simulink model "HLB_trp"  (R2019b)
settings: Solver=FixedStepDiscrete  StartTime=0.0  StopTime=1000.0  FixedStep=0.01  RelTol=1e-3
InitFcn:
  | %load('20220808.mat')
libraries: driver_model_library x6, simulink x3, CarMaker4SL x1
settings Model: Creator=DOT1BP  LastModifiedBy=DOT1BP
settings ModelReferenceCC: ModelReferenceNumInstancesAllowed=Single

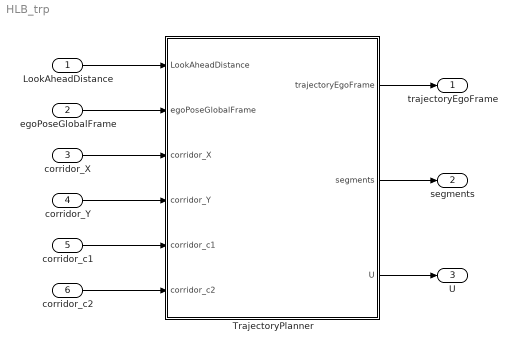
== system HLB_trp ==
  LookAheadDistance : Inport
  egoPoseGlobalFrame : Inport  Port=2  PortDimensions=[3,1]
  corridor_X : Inport  Port=3  PortDimensions=[301,1]
  corridor_Y : Inport  Port=4  PortDimensions=[301,1]
  corridor_c1 : Inport  Port=5  PortDimensions=[301,1]
  corridor_c2 : Inport  Port=6  PortDimensions=[301,1]
  TrajectoryPlanner : Subsystem
  trajectoryEgoFrame : Outport
  segments : Outport  Port=2
  U : Outport  Port=3
  wires:
  TrajectoryPlanner/1(trajectoryEgoFrame) -> trajectoryEgoFrame/1
  TrajectoryPlanner/2(segments) -> segments/1
  TrajectoryPlanner/3(U) -> U/1
  corridor_c2/1 -> TrajectoryPlanner/6(corridor_c2)
  corridor_c1/1 -> TrajectoryPlanner/5(corridor_c1)
  corridor_Y/1 -> TrajectoryPlanner/4(corridor_Y)
  corridor_X/1 -> TrajectoryPlanner/3(corridor_X)
  egoPoseGlobalFrame/1 -> TrajectoryPlanner/2(egoPoseGlobalFrame)
  LookAheadDistance/1 -> TrajectoryPlanner/1("LookAheadDistance ")

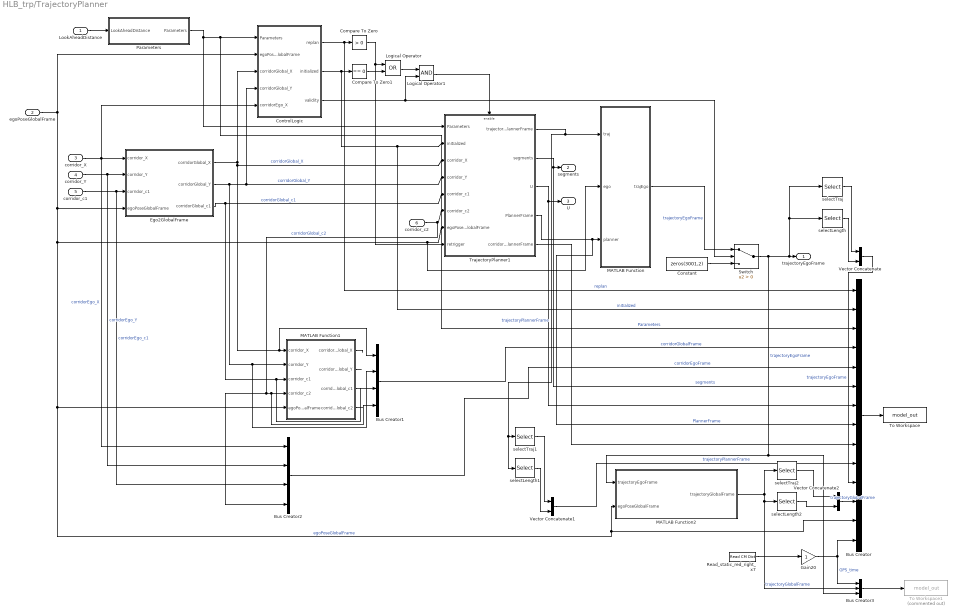
== system HLB_trp/TrajectoryPlanner ==
  "LookAheadDistance " : Inport
  egoPoseGlobalFrame : Inport  Port=2
  corridor_X : Inport  Port=3
  corridor_Y : Inport  Port=4
  corridor_c1 : Inport  Port=5
  corridor_c2 : Inport  Port=6
  Bus Creator : BusCreator  Inputs=14
  Bus Creator1 : BusCreator  Inputs=4
  Bus Creator2 : BusCreator  Inputs=4
  Bus Creator3 : BusCreator  Inputs=3
  Compare To Zero : simulink/Logic and Bit Operations/Compare To Zero  relop=>  OutDataTypeStr=boolean
  Compare To Zero1 : simulink/Logic and Bit Operations/Compare To Zero  relop===  OutDataTypeStr=boolean
  Constant : Constant  Value=zeros(3001,2)
  ControlLogic : Subsystem
  Ego2GlobalFrame : MATLAB Function  TreatAsAtomicUnit=on
  Gain20 : Gain
  Logical Operator : Logic  Operator=OR  AllPortsSameDT=off  OutDataTypeStr=boolean
  Logical Operator1 : Logic  AllPortsSameDT=off  OutDataTypeStr=boolean
  MATLAB Function : MATLAB Function  TreatAsAtomicUnit=on
  MATLAB Function1 : MATLAB Function  TreatAsAtomicUnit=on
  MATLAB Function2 : MATLAB Function  TreatAsAtomicUnit=on
  Parameters : Subsystem
  Read_static_red_right_x7 : CarMaker4SL/Read CM Dict  xname=Time.Global  xsync=off
  Switch : Switch  Criteria=u2 > Threshold
  To Workspace : ToWorkspace  VariableName=model_out  SaveFormat=Timeseries  SampleTime=-1
  To Workspace1 : ToWorkspace  Commented=on  VariableName=model_out  SaveFormat=Timeseries  SampleTime=-1
  TrajectoryPlanner1 : Subsystem
  Vector Concatenate : Concatenate  Mode=Multidimensional array
  Vector Concatenate1 : Concatenate  Mode=Multidimensional array
  Vector Concatenate2 : Concatenate  Mode=Multidimensional array
  selectLength : Selector  NumberOfDimensions=2  InputPortWidth=3  IndexOptions=Index vector (dialog),Index vector (dialog)  Indices=[3001],[1 2]  OutputSizes=1,1
  selectLength1 : Selector  NumberOfDimensions=2  InputPortWidth=3  IndexOptions=Index vector (dialog),Index vector (dialog)  Indices=[3001],[1 2]  OutputSizes=1,1
  selectLength2 : Selector  NumberOfDimensions=2  InputPortWidth=3  IndexOptions=Index vector (dialog),Index vector (dialog)  Indices=[3001],[1 2]  OutputSizes=1,1
  selectTraj : Selector  NumberOfDimensions=2  InputPortWidth=3  IndexOptions=Index vector (dialog),Index vector (dialog)  Indices=linspace(1,300,300),[1 2]  OutputSizes=1,1
  selectTraj1 : Selector  NumberOfDimensions=2  InputPortWidth=3  IndexOptions=Index vector (dialog),Index vector (dialog)  Indices=linspace(1,300,300),[1 2]  OutputSizes=1,1
  selectTraj2 : Selector  NumberOfDimensions=2  InputPortWidth=3  IndexOptions=Index vector (dialog),Index vector (dialog)  Indices=linspace(1,300,300),[1 2]  OutputSizes=1,1
  trajectoryEgoFrame : Outport
  segments : Outport  Port=2
  U : Outport  Port=3
  wires:
  ControlLogic/2(initialized) -> TrajectoryPlanner1/2(initialized), Bus Creator/2, Compare To Zero1/1  "initialized"
  TrajectoryPlanner1/3(U) -> U/1, Bus Creator/7
  Compare To Zero1/1 -> Logical Operator/2
  ControlLogic/1(replan) -> Bus Creator/1, Compare To Zero/1  "replan"
  "LookAheadDistance "/1 -> Parameters/1(LookAheadDistance)
  TrajectoryPlanner1/2(segments) -> Bus Creator/6, segments/1  "segments"
  Compare To Zero/1 -> TrajectoryPlanner1/8(retrigger), Logical Operator/1
  Parameters/1("Parameters ") -> ControlLogic/1(Parameters), Bus Creator/3, TrajectoryPlanner1/1("Parameters ")  "Parameters"
  corridor_c2/1 -> MATLAB Function1/4(corridor_c2), Bus Creator1/4, Bus Creator2/4, TrajectoryPlanner1/6(corridor_c2)  "corridorGlobal_c2"
  MATLAB Function/1(trajEgo) -> Switch/1  "trajectoryEgoFrame"
  TrajectoryPlanner1/1(trajectoryPlannerFrame) -> selectLength1/1, selectTraj1/1, MATLAB Function/1(traj)  "trajectoryPlannerFrame"
  TrajectoryPlanner1/4(PlannerFrame) -> MATLAB Function/3(planner), Bus Creator/8  "PlannerFrame"
  corridor_X/1 -> ControlLogic/5(corridorEgo_X), Ego2GlobalFrame/1(corridor_X), Bus Creator2/1  "corridorEgo_X"
  corridor_Y/1 -> Ego2GlobalFrame/2(corridor_Y), Bus Creator2/2  "corridorEgo_Y"
  corridor_c1/1 -> Bus Creator2/3, Ego2GlobalFrame/3(corridor_c1)  "corridorEgo_c1"
  Ego2GlobalFrame/1(corridorGlobal_X) -> TrajectoryPlanner1/3(corridor_X), Bus Creator1/1, MATLAB Function1/1(corridor_X), ControlLogic/3(corridorGlobal_X)  "corridorGlobal_X"
  Ego2GlobalFrame/2(corridorGlobal_Y) -> MATLAB Function1/2(corridor_Y), Bus Creator1/2, TrajectoryPlanner1/4(corridor_Y), ControlLogic/4(corridorGlobal_Y)  "corridorGlobal_Y"
  Ego2GlobalFrame/3(corridorGlobal_c1) -> MATLAB Function1/3(corridor_c1), Bus Creator1/3, TrajectoryPlanner1/5(corridor_c1)  "corridorGlobal_c1"
  egoPoseGlobalFrame/1 -> ControlLogic/2(egoPoseGlobalFrame), Bus Creator/13, MATLAB Function2/2(egoPoseGlobalFrame), MATLAB Function1/5(egoPoseGlobalFrame), TrajectoryPlanner1/7(egoPoseGlobalFrame), MATLAB Function/2(ego), Ego2GlobalFrame/4(egoPoseGlobalFrame)  "egoPoseGlobalFrame"
  Logical Operator/1 -> Logical Operator1/1
  Logical Operator1/1 -> TrajectoryPlanner1/Enable
  Switch/1 -> selectLength/1, selectTraj/1, trajectoryEgoFrame/1, Bus Creator3/3, MATLAB Function2/1(trajectoryEgoFrame)  "trajectoryEgoFrame"
  Constant/1 -> Switch/3
  Bus Creator/1 -> To Workspace/1
  MATLAB Function1/1(corridorGlobal_X) -> ?
  MATLAB Function1/2(corridorGlobal_Y) -> ?
  MATLAB Function1/3(corridorGlobal_c1) -> ?
  MATLAB Function1/4(corridorGlobal_c2) -> ?
  Bus Creator1/1 -> Bus Creator/4  "corridorGlobalFrame"
  Bus Creator2/1 -> Bus Creator/5  "corridorEgoFrame"
  TrajectoryPlanner1/5(corridorPlannerFrame) -> Bus Creator/9
  MATLAB Function2/1(trajectoryGlobalFrame) -> selectTraj2/1, selectLength2/1, Bus Creator3/2  "trajectoryGlobalFrame"
  Read_static_red_right_x7/1 -> Gain20/1
  Gain20/1 -> Bus Creator/14, Bus Creator3/1  "GPS_time"
  Bus Creator3/1 -> To Workspace1/1
  selectTraj/1 -> Vector Concatenate/1
  selectLength/1 -> Vector Concatenate/2
  ControlLogic/3(validity) -> Logical Operator1/2, Switch/2
  Vector Concatenate/1 -> Bus Creator/11  "trajectoryEgoFrame"
  selectTraj1/1 -> Vector Concatenate1/1
  selectLength1/1 -> Vector Concatenate1/2
  Vector Concatenate1/1 -> Bus Creator/10  "trajectoryPlannerFrame"
  selectTraj2/1 -> Vector Concatenate2/1
  selectLength2/1 -> Vector Concatenate2/2
  Vector Concatenate2/1 -> Bus Creator/12  "trajectoryGlobalFrame"

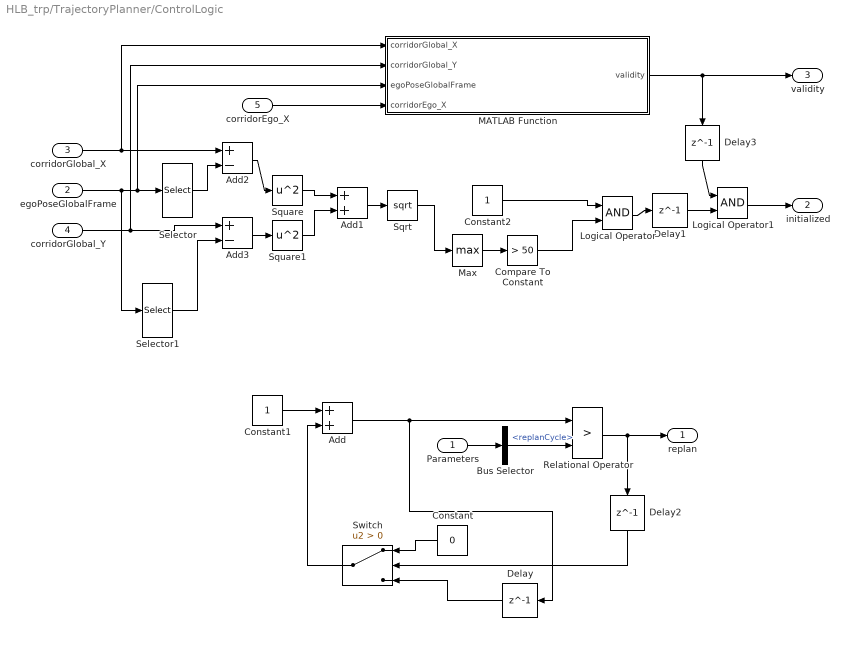
== system HLB_trp/TrajectoryPlanner/ControlLogic ==
  Parameters : Inport
  egoPoseGlobalFrame : Inport  Port=2
  corridorGlobal_X : Inport  Port=3
  corridorGlobal_Y : Inport  Port=4
  corridorEgo_X : Inport  Port=5
  Add : Sum
  Add1 : Sum
  Add2 : Sum  Inputs=+-
  Add3 : Sum  Inputs=+-
  Bus Selector : BusSelector  OutputSignals=replanCycle
  Compare To Constant : simulink/Logic and Bit Operations/Compare To Constant  relop=>  const=50  OutDataTypeStr=boolean
  Constant : Constant  Value=0
  Constant1 : Constant
  Constant2 : Constant
  Delay{,1..3} (4 alike) : Delay  DelayLength=1  InitialCondition=0
  Logical Operator : Logic  AllPortsSameDT=off  OutDataTypeStr=boolean
  Logical Operator1 : Logic  AllPortsSameDT=off  OutDataTypeStr=boolean
  MATLAB Function : MATLAB Function  TreatAsAtomicUnit=on
  Max : MinMax  Function=max
  Relational Operator : RelationalOperator  Operator=>  OutDataTypeStr=boolean  RndMeth=Simplest
  Selector : Selector  InputPortWidth=3  IndexOptions=Index vector (dialog)  Indices=[1]  OutputSizes=1
  Selector1 : Selector  InputPortWidth=3  IndexOptions=Index vector (dialog)  Indices=[2]  OutputSizes=1
  Sqrt : Sqrt  SaturateOnIntegerOverflow=on
  Square : Math  Operator=square  SignedPower=off  SaturateOnIntegerOverflow=on
  Square1 : Math  Operator=square  SignedPower=off  SaturateOnIntegerOverflow=on
  Switch : Switch  Criteria=u2 > Threshold
  replan : Outport
  initialized : Outport  Port=2
  validity : Outport  Port=3
  wires:
  Add/1 -> Relational Operator/1, Delay/1
  Parameters/1 -> Bus Selector/1
  Bus Selector/1 -> Relational Operator/2  "<replanCycle>"
  Relational Operator/1 -> Delay2/1, replan/1
  Constant/1 -> Switch/1
  Delay/1 -> Switch/3
  Switch/1 -> Add/2
  Constant1/1 -> Add/1
  Logical Operator/1 -> Delay1/1
  Constant2/1 -> Logical Operator/1
  Square/1 -> Add1/1
  Square1/1 -> Add1/2
  Add1/1 -> Sqrt/1
  Sqrt/1 -> Max/1
  Compare To Constant/1 -> Logical Operator/2
  Max/1 -> Compare To Constant/1
  Delay2/1 -> Switch/2
  egoPoseGlobalFrame/1 -> Selector/1, MATLAB Function/3(egoPoseGlobalFrame), Selector1/1
  corridorGlobal_X/1 -> Add2/1, MATLAB Function/1(corridorGlobal_X)
  Selector/1 -> Add2/2
  Add2/1 -> Square/1
  Add3/1 -> Square1/1
  corridorGlobal_Y/1 -> Add3/1, MATLAB Function/2(corridorGlobal_Y)
  Selector1/1 -> Add3/2
  MATLAB Function/1(validity) -> Delay3/1, validity/1
  Delay1/1 -> Logical Operator1/2
  Logical Operator1/1 -> initialized/1
  Delay3/1 -> Logical Operator1/1
  corridorEgo_X/1 -> MATLAB Function/4(corridorEgo_X)

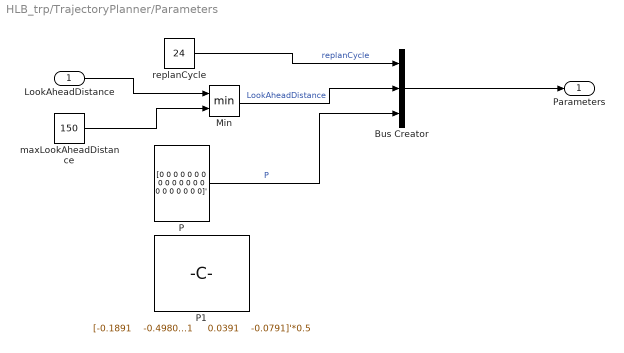
== system HLB_trp/TrajectoryPlanner/Parameters ==
  LookAheadDistance : Inport
  Bus Creator : BusCreator  Inputs=3
  Min : MinMax  Inputs=2
  P : Constant  Value=[0 0 0 0 0 0 0 0 0 0 0 0 0 0 0 0 0 0 0 0 0]'
  P1 : Constant  Value=|
      | [-0.1891
      |    -0.4980
      |     0.6295
      |     0.5723
      |     0.9711
      |    -0.8867
      |    -0.2526
      |    -0.3461
      |     0.3919
      |    -0.0105
      |     0.0010
      |     0.0183
      |     0.0167
      |    -0.0047
      |     0.0494
      |    -0.0250
      |     0.0333
      |    -0.0235
      |     0.0681
      |     0.0391
      |    -0.0791]'*0.5
  maxLookAheadDistance : Constant  Value=150
  replanCycle : Constant  Value=24
  "Parameters " : Outport
  wires:
  Min/1 -> Bus Creator/2  "LookAheadDistance"
  Bus Creator/1 -> "Parameters "/1
  maxLookAheadDistance/1 -> Min/2
  LookAheadDistance/1 -> Min/1
  replanCycle/1 -> Bus Creator/1  "replanCycle"
  P/1 -> Bus Creator/3  "P"

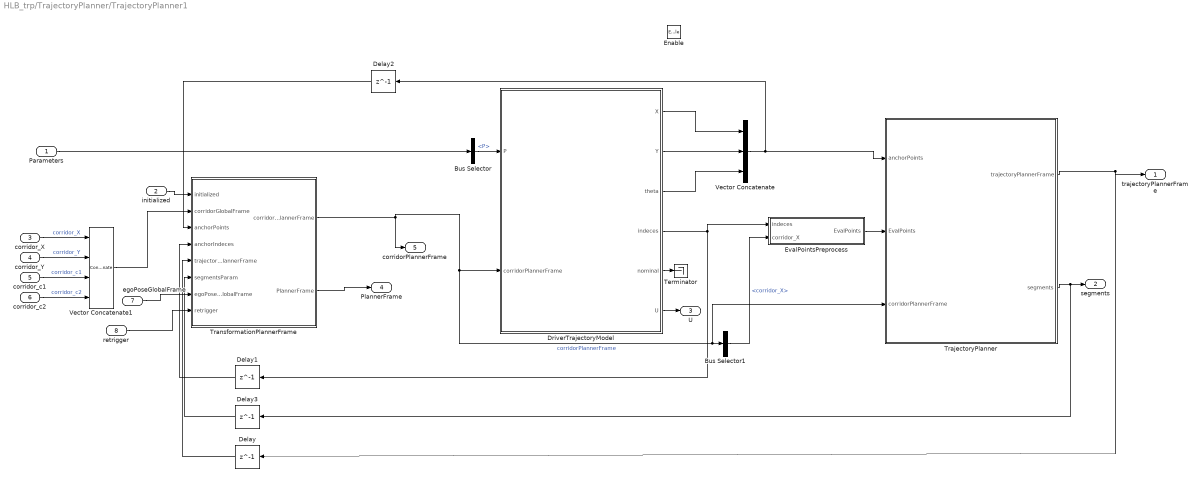
== system HLB_trp/TrajectoryPlanner/TrajectoryPlanner1 ==
  "Parameters " : Inport
  initialized : Inport  Port=2
  corridor_X : Inport  Port=3
  corridor_Y : Inport  Port=4
  corridor_c1 : Inport  Port=5
  corridor_c2 : Inport  Port=6
  egoPoseGlobalFrame : Inport  Port=7
  retrigger : Inport  Port=8
  Enable : EnablePort
  Bus Selector : BusSelector  OutputSignals=P
  Bus Selector1 : BusSelector  OutputSignals=corridor_X
  Delay : Delay  DelayLength=1  InitialCondition=zeros(3001,2)
  Delay1 : Delay  DelayLength=1  InitialCondition=zeros(4,1)
  Delay2 : Delay  DelayLength=1  InitialCondition=zeros(12,1)
  Delay3 : Delay  DelayLength=1  InitialCondition=zeros(3,6)
  DriverTrajectoryModel : Subsystem
  EvalPointsPreprocess : Subsystem
  Terminator : Terminator
  TrajectoryPlanner : Subsystem
  TransformationPlannerFrame : Subsystem
  Vector Concatenate : Concatenate  NumInputs=3
  Vector Concatenate1 : Concatenate  NumInputs=4  Mode=Multidimensional array  ConcatenateDimension=2
  trajectoryPlannerFrame : Outport
  segments : Outport  Port=2
  U : Outport  Port=3
  PlannerFrame : Outport  Port=4
  corridorPlannerFrame : Outport  Port=5
  wires:
  DriverTrajectoryModel/3(theta) -> Vector Concatenate/3
  EvalPointsPreprocess/1(EvalPoints) -> TrajectoryPlanner/2(EvalPoints)
  DriverTrajectoryModel/1(X) -> Vector Concatenate/1
  DriverTrajectoryModel/2(Y) -> Vector Concatenate/2
  DriverTrajectoryModel/5(nominal) -> Terminator/1
  Vector Concatenate/1 -> Delay2/1, TrajectoryPlanner/1(anchorPoints)
  DriverTrajectoryModel/4(indeces) -> Delay1/1, EvalPointsPreprocess/1(indeces)
  TrajectoryPlanner/1(trajectoryPlannerFrame) -> trajectoryPlannerFrame/1, Delay/1
  DriverTrajectoryModel/6(U) -> U/1
  TrajectoryPlanner/2(segments) -> segments/1, Delay3/1
  "Parameters "/1 -> Bus Selector/1
  Bus Selector/1 -> DriverTrajectoryModel/1(P)  "<P>"
  TransformationPlannerFrame/1(corridorPlannerFrame) -> TrajectoryPlanner/3(corridorPlannerFrame), Bus Selector1/1, DriverTrajectoryModel/2(corridorPlannerFrame), corridorPlannerFrame/1  "corridorPlannerFrame"
  initialized/1 -> TransformationPlannerFrame/1(initialized)
  Delay/1 -> TransformationPlannerFrame/5(trajectoryPreviousPlannerFrame)
  corridor_c1/1 -> Vector Concatenate1/3  "corridor_c1"
  corridor_X/1 -> Vector Concatenate1/1  "corridor_X"
  corridor_Y/1 -> Vector Concatenate1/2  "corridor_Y"
  corridor_c2/1 -> Vector Concatenate1/4  "corridor_c2"
  Vector Concatenate1/1 -> TransformationPlannerFrame/2(corridorGlobalFrame)
  Delay1/1 -> TransformationPlannerFrame/4(anchorIndeces)
  Delay2/1 -> TransformationPlannerFrame/3(anchorPoints)
  TransformationPlannerFrame/2(PlannerFrame) -> PlannerFrame/1
  Delay3/1 -> TransformationPlannerFrame/6(segmentsParam)
  egoPoseGlobalFrame/1 -> TransformationPlannerFrame/7(egoPoseGlobalFrame)
  Bus Selector1/1 -> EvalPointsPreprocess/2(corridor_X)  "<corridor_X>"
  retrigger/1 -> TransformationPlannerFrame/8(retrigger)

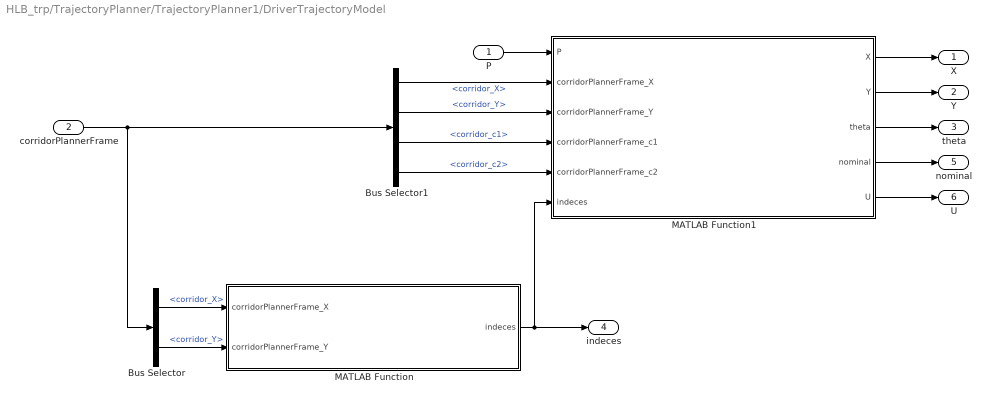
== system HLB_trp/TrajectoryPlanner/TrajectoryPlanner1/DriverTrajectoryModel ==
  P : Inport
  corridorPlannerFrame : Inport  Port=2
  Bus Selector : BusSelector  OutputSignals=corridor_X,corridor_Y
  Bus Selector1 : BusSelector  OutputSignals=corridor_X,corridor_Y,corridor_c1,corridor_c2
  MATLAB Function : MATLAB Function  TreatAsAtomicUnit=on
  MATLAB Function1 : MATLAB Function  TreatAsAtomicUnit=on
  X : Outport
  Y : Outport  Port=2
  theta : Outport  Port=3
  indeces : Outport  Port=4
  nominal : Outport  Port=5
  U : Outport  Port=6
  wires:
  MATLAB Function/1(indeces) -> indeces/1, MATLAB Function1/6(indeces)
  P/1 -> MATLAB Function1/1(P)
  MATLAB Function1/1(X) -> X/1
  MATLAB Function1/2(Y) -> Y/1
  MATLAB Function1/3(theta) -> theta/1
  MATLAB Function1/4(nominal) -> nominal/1
  MATLAB Function1/5(U) -> U/1
  corridorPlannerFrame/1 -> Bus Selector/1, Bus Selector1/1
  Bus Selector/1 -> MATLAB Function/1(corridorPlannerFrame_X)  "<corridor_X>"
  Bus Selector/2 -> MATLAB Function/2(corridorPlannerFrame_Y)  "<corridor_Y>"
  Bus Selector1/1 -> MATLAB Function1/2(corridorPlannerFrame_X)  "<corridor_X>"
  Bus Selector1/2 -> MATLAB Function1/3(corridorPlannerFrame_Y)  "<corridor_Y>"
  Bus Selector1/3 -> MATLAB Function1/4(corridorPlannerFrame_c1)  "<corridor_c1>"
  Bus Selector1/4 -> MATLAB Function1/5(corridorPlannerFrame_c2)  "<corridor_c2>"

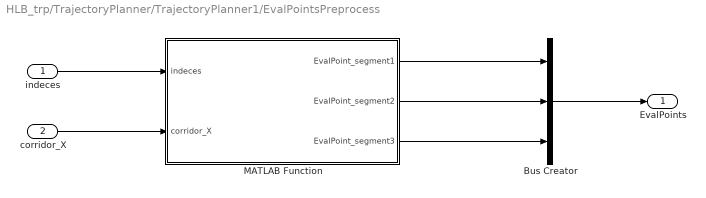
== system HLB_trp/TrajectoryPlanner/TrajectoryPlanner1/EvalPointsPreprocess ==
  indeces : Inport
  corridor_X : Inport  Port=2
  Bus Creator : BusCreator  Inputs=3
  MATLAB Function : MATLAB Function  TreatAsAtomicUnit=on
  EvalPoints : Outport
  wires:
  indeces/1 -> MATLAB Function/1(indeces)
  corridor_X/1 -> MATLAB Function/2(corridor_X)
  MATLAB Function/1(EvalPoint_segment1) -> Bus Creator/1
  MATLAB Function/2(EvalPoint_segment2) -> Bus Creator/2
  MATLAB Function/3(EvalPoint_segment3) -> Bus Creator/3
  Bus Creator/1 -> EvalPoints/1

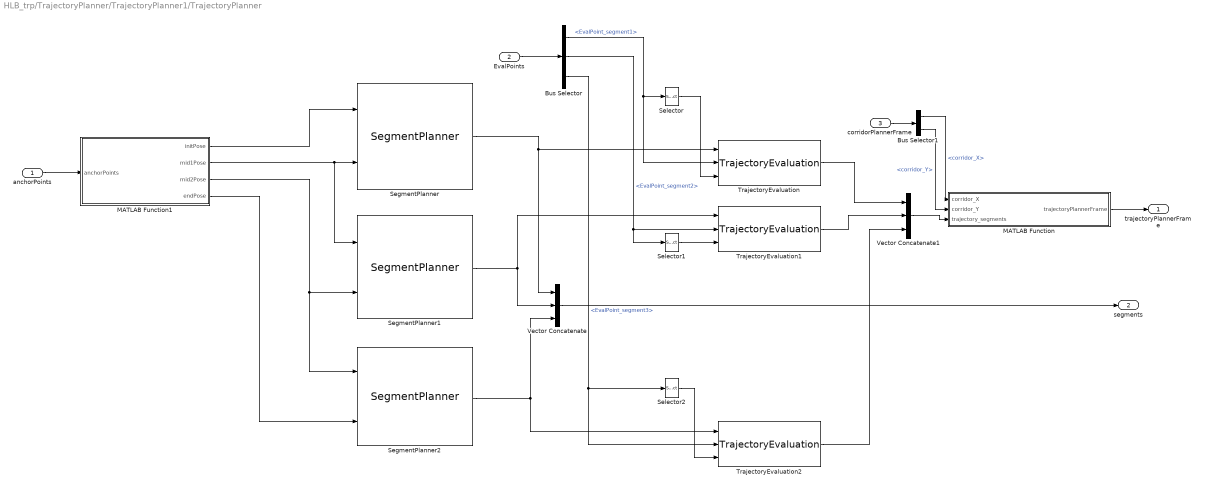
== system HLB_trp/TrajectoryPlanner/TrajectoryPlanner1/TrajectoryPlanner ==
  anchorPoints : Inport
  EvalPoints : Inport  Port=2
  corridorPlannerFrame : Inport  Port=3
  Bus Selector : BusSelector  OutputSignals=EvalPoint_segment1,EvalPoint_segment2,EvalPoint_segment3
  Bus Selector1 : BusSelector  OutputSignals=corridor_X,corridor_Y
  MATLAB Function : MATLAB Function  TreatAsAtomicUnit=on
  MATLAB Function1 : MATLAB Function  TreatAsAtomicUnit=on
  SegmentPlanner : driver_model_library/SegmentPlanner  SystemSampleTime=-1  Latency=0  AutoFrameSizeCalculation=off
  SegmentPlanner1 : driver_model_library/SegmentPlanner  SystemSampleTime=-1  Latency=0  AutoFrameSizeCalculation=off
  SegmentPlanner2 : driver_model_library/SegmentPlanner  SystemSampleTime=-1  Latency=0  AutoFrameSizeCalculation=off
  Selector : Selector  InputPortWidth=1001  IndexOptions=Index vector (dialog)  Indices=1001  OutputSizes=1
  Selector1 : Selector  InputPortWidth=1001  IndexOptions=Index vector (dialog)  Indices=1001  OutputSizes=1
  Selector2 : Selector  InputPortWidth=1001  IndexOptions=Index vector (dialog)  Indices=1001  OutputSizes=1
  TrajectoryEvaluation : driver_model_library/TrajectoryEvaluation  SystemSampleTime=-1  Latency=0  AutoFrameSizeCalculation=off
  TrajectoryEvaluation1 : driver_model_library/TrajectoryEvaluation  SystemSampleTime=-1  Latency=0  AutoFrameSizeCalculation=off
  TrajectoryEvaluation2 : driver_model_library/TrajectoryEvaluation  SystemSampleTime=-1  Latency=0  AutoFrameSizeCalculation=off
  Vector Concatenate : Concatenate  NumInputs=3  Mode=Multidimensional array
  Vector Concatenate1 : Concatenate  NumInputs=3  Mode=Multidimensional array
  trajectoryPlannerFrame : Outport
  segments : Outport  Port=2
  wires:
  anchorPoints/1 -> MATLAB Function1/1(anchorPoints)
  MATLAB Function1/1(initPose) -> SegmentPlanner/1
  MATLAB Function1/2(mid1Pose) -> SegmentPlanner/2, SegmentPlanner1/1
  MATLAB Function1/3(mid2Pose) -> SegmentPlanner1/2, SegmentPlanner2/1
  MATLAB Function1/4(endPose) -> SegmentPlanner2/2
  SegmentPlanner/1 -> TrajectoryEvaluation/1, Vector Concatenate/1
  SegmentPlanner1/1 -> TrajectoryEvaluation1/1, Vector Concatenate/2
  SegmentPlanner2/1 -> Vector Concatenate/3, TrajectoryEvaluation2/1
  Vector Concatenate/1 -> segments/1
  TrajectoryEvaluation/1 -> Vector Concatenate1/1
  TrajectoryEvaluation1/1 -> Vector Concatenate1/2
  TrajectoryEvaluation2/1 -> Vector Concatenate1/3
  EvalPoints/1 -> Bus Selector/1
  Bus Selector/1 -> TrajectoryEvaluation/2, Selector/1  "<EvalPoint_segment1>"
  Bus Selector/2 -> Selector1/1, TrajectoryEvaluation1/2  "<EvalPoint_segment2>"
  Bus Selector/3 -> Selector2/1, TrajectoryEvaluation2/2  "<EvalPoint_segment3>"
  Selector/1 -> TrajectoryEvaluation/3
  Selector1/1 -> TrajectoryEvaluation1/3
  Selector2/1 -> TrajectoryEvaluation2/3
  Vector Concatenate1/1 -> MATLAB Function/3(trajectory_segments)
  MATLAB Function/1(trajectoryPlannerFrame) -> trajectoryPlannerFrame/1
  corridorPlannerFrame/1 -> Bus Selector1/1
  Bus Selector1/2 -> MATLAB Function/2(corridor_Y)  "<corridor_Y>"
  Bus Selector1/1 -> MATLAB Function/1(corridor_X)  "<corridor_X>"

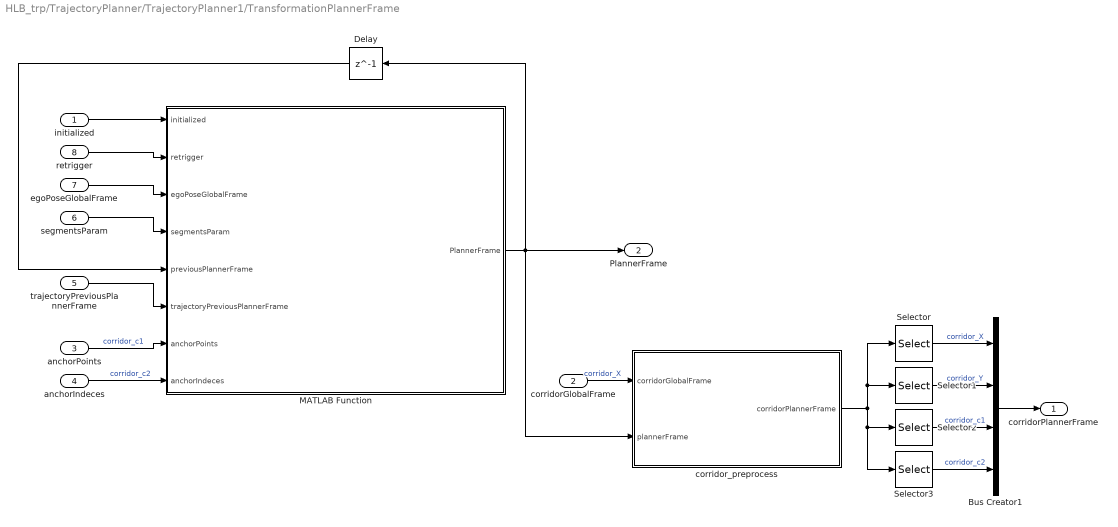
== system HLB_trp/TrajectoryPlanner/TrajectoryPlanner1/TransformationPlannerFrame ==
  initialized : Inport
  corridorGlobalFrame : Inport  Port=2
  anchorPoints : Inport  Port=3
  anchorIndeces : Inport  Port=4
  trajectoryPreviousPlannerFrame : Inport  Port=5
  segmentsParam : Inport  Port=6
  egoPoseGlobalFrame : Inport  Port=7
  retrigger : Inport  Port=8
  Bus Creator1 : BusCreator  Inputs=4
  Delay : Delay  DelayLength=1  InitialCondition=zeros(3,1)
  MATLAB Function : MATLAB Function  TreatAsAtomicUnit=on
  Selector : Selector  NumberOfDimensions=2  InputPortWidth=3  IndexOptions=Select all,Index vector (dialog)  Indices=[1 3],1  OutputSizes=1,1
  Selector1 : Selector  NumberOfDimensions=2  InputPortWidth=3  IndexOptions=Select all,Index vector (dialog)  Indices=[1 3],2  OutputSizes=1,1
  Selector2 : Selector  NumberOfDimensions=2  InputPortWidth=3  IndexOptions=Select all,Index vector (dialog)  Indices=[1 3],3  OutputSizes=1,1
  Selector3 : Selector  NumberOfDimensions=2  InputPortWidth=3  IndexOptions=Select all,Index vector (dialog)  Indices=[1 3],4  OutputSizes=1,1
  corridor_preprocess : MATLAB Function  TreatAsAtomicUnit=on
  corridorPlannerFrame : Outport
  PlannerFrame : Outport  Port=2
  wires:
  Bus Creator1/1 -> corridorPlannerFrame/1
  corridor_preprocess/1(corridorPlannerFrame) -> Selector3/1, Selector2/1, Selector1/1, Selector/1
  Selector/1 -> Bus Creator1/1  "corridor_X"
  Selector1/1 -> Bus Creator1/2  "corridor_Y"
  Selector2/1 -> Bus Creator1/3  "corridor_c1"
  Selector3/1 -> Bus Creator1/4  "corridor_c2"
  trajectoryPreviousPlannerFrame/1 -> MATLAB Function/6(trajectoryPreviousPlannerFrame)
  MATLAB Function/1(PlannerFrame) -> PlannerFrame/1, Delay/1, corridor_preprocess/2(plannerFrame)
  Delay/1 -> MATLAB Function/5(previousPlannerFrame)
  anchorPoints/1 -> MATLAB Function/7(anchorPoints)  "corridor_c1"
  anchorIndeces/1 -> MATLAB Function/8(anchorIndeces)  "corridor_c2"
  corridorGlobalFrame/1 -> corridor_preprocess/1(corridorGlobalFrame)  "corridor_X"
  initialized/1 -> MATLAB Function/1(initialized)
  segmentsParam/1 -> MATLAB Function/4(segmentsParam)
  egoPoseGlobalFrame/1 -> MATLAB Function/3(egoPoseGlobalFrame)
  retrigger/1 -> MATLAB Function/2(retrigger)

== matlab function HLB_trp/TrajectoryPlanner/TrajectoryPlanner1/TrajectoryPlanner/MATLAB Function1 ==
  data: anchorPoints input; initPose output; mid1Pose output; mid2Pose output; endPose output
function [initPose, mid1Pose, mid2Pose, endPose] = preprocess_poses(anchorPoints)

initPose = anchorPoints(1:4:end);
mid1Pose = anchorPoints(2:4:end);
mid2Pose = anchorPoints(3:4:end);
endPose = anchorPoints(4:4:end);

end

== matlab function HLB_trp/TrajectoryPlanner/TrajectoryPlanner1/EvalPointsPreprocess/MATLAB Function ==
  data: indeces input; EvalPoint_segment1 output; corridor_X input; EvalPoint_segment2 output; EvalPoint_segment3 output
function [EvalPoint_segment1, EvalPoint_segment2, EvalPoint_segment3] = selectEvalPoints(indeces, corridor_X)

n_1 = indeces(2) - 1;
n_2 = indeces(3) - indeces(2);
n_3 = indeces(4) - indeces(3) + 1;

EvalPoint_segment1 = zeros(1001,1);
EvalPoint_segment2 = zeros(1001,1);
EvalPoint_segment3 = zeros(1001,1);


EvalPoint_segment1(1:n_1,1) = corridor_X(1:indeces(2)-1,1);
EvalPoint_segment2(1:n_2,1) = corridor_X(indeces(2):indeces(3)-1,1);
EvalPoint_segment3(1:n_3,1) = corridor_X(indeces(3):indeces(4),1);

EvalPoint_segment1(1001,1) = n_1;
EvalPoint_segment2(1001,1) = n_2;
EvalPoint_segment3(1001,1) = n_3;

end

== matlab function HLB_trp/TrajectoryPlanner/TrajectoryPlanner1/DriverTrajectoryModel/MATLAB Function ==
  data: corridorPlannerFrame_X input; indeces output; corridorPlannerFrame_Y input
function indeces  = node_point_model(corridorPlannerFrame_X, corridorPlannerFrame_Y)
% test
n = corridorPlannerFrame_X(301);
corridorPlannerFrame_X = corridorPlannerFrame_X(1:n,1);
corridorPlannerFrame_Y = corridorPlannerFrame_Y(1:n,1);
% delete afterwards
% preprocess bc of test case
non_negative_index = 0;
[non_negative_index] = find(corridorPlannerFrame_X > 0,1);
non_negative_index = non_negative_index(1);
% remove slicing after finished with simulation cases
P = [0; 26.59; 96.91];
n = size(corridorPlannerFrame_X(non_negative_index:end),1);
lengths = zeros(n,1);

lengths(:,1) = (corridorPlannerFrame_X(non_negative_index:end).^2+corridorPlannerFrame_Y(non_negative_index:end).^2).^0.5;

minStepDist = 10; % in meters
indeces = zeros(4,1);
indeces(1) = 1;

L = zeros(1,4);

L(2) = min(lengths(end)-3*minStepDist,max(minStepDist,P(1)));
L(3) = min(lengths(end)-2*minStepDist,max(L(2)+minStepDist,L(2)+P(2)));
L(4) = min(lengths(end)-minStepDist,max(L(3)+minStepDist,L(3)+P(3)));

index_1 = 0;
index_2 = 0;
index_3 = 0;

[index_1] = find(lengths>=L(2),1);
indeces(2) = index_1;
    
[index_2] = find(lengths>=L(3),1);
indeces(3) = index_2;

[index_3] = find(lengths>=L(4),1);
indeces(4) = min(n,index_3);
end

== matlab function HLB_trp/TrajectoryPlanner/TrajectoryPlanner1/DriverTrajectoryModel/MATLAB Function1 ==
  data: P input; X output; corridorPlannerFrame_X input; corridorPlannerFrame_Y input; corridorPlannerFrame_c1 input; corridorPlannerFrame_c2 input; indeces input; Y output; theta output; nominal output; U output
function [X, Y, theta, nominal, U] = driver_model_planner(P, corridorPlannerFrame_X, corridorPlannerFrame_Y, corridorPlannerFrame_c1, corridorPlannerFrame_c2, indeces)
%test
n = corridorPlannerFrame_X(301);
corridorPlannerFrame_X = corridorPlannerFrame_X(1:n,1);
corridorPlannerFrame_Y = corridorPlannerFrame_Y(1:n,1);
corridorPlannerFrame_c1 = corridorPlannerFrame_c1(1:n,1);
corridorPlannerFrame_c2 = corridorPlannerFrame_c2(1:n,1);
%delete afterwards
% preprocess bc of test case
non_negative_index = 0;
[non_negative_index] = find(corridorPlannerFrame_X >= 0,1);
non_negative_index = non_negative_index(1);
corridorPlannerFrame_X = corridorPlannerFrame_X(non_negative_index:end);
corridorPlannerFrame_Y = corridorPlannerFrame_Y(non_negative_index:end);
corridorPlannerFrame_c1 = corridorPlannerFrame_c1(non_negative_index:end);
corridorPlannerFrame_c2 = corridorPlannerFrame_c2(non_negative_index:end);
% remove slicing after finished with simulation cases
P1 = reshape(P(1:21,1),3,7);

X = zeros(4,1);
Y = zeros(4,1);
theta = zeros(4,1);

X_nominal = corridorPlannerFrame_X(indeces);
Y_nominal = corridorPlannerFrame_Y(indeces);
theta_nominal = corridorPlannerFrame_c1(indeces); % orientation in radian
kappa_nominal = zeros(length(indeces)-1, 1);
dkappa_nominal = zeros(length(indeces)-1, 1);

for j=1:length(indeces)-1
    kappa_nominal(j,1) = mean(corridorPlannerFrame_c2(indeces(j):indeces(j+1)));
end

dkappa_vector = zeros(length(corridorPlannerFrame_X),1);
dkappa_vector(2:end) = diff(corridorPlannerFrame_c2)./diff(corridorPlannerFrame_X);
dkappa_vector(1) = diff(corridorPlannerFrame_c2(1:2))/diff(corridorPlannerFrame_X(1:2));
dkappa_vector = movmean(dkappa_vector,50);

% extra corridor information
nominal = [X_nominal; Y_nominal; theta_nominal];

dkappa_nominal = dkappa_vector(indeces);


U = zeros(length(indeces)-1+length(indeces), 1);
U(1:length(indeces)-1,1) = kappa_nominal;
U(length(indeces):end,1) = dkappa_nominal;

% scaling of the predictor variables
kappa_lim = 0.001;
dkappa_lim = 1e-5;
U_lim = [ones(3,1)*kappa_lim; ones(4,1)*dkappa_lim];
U = U./U_lim;

% the ouput of the model is the linear combination of predictor variables
% P parameter matrix is given to the model.
x = P1*U;
x(1:3) = x(1:3);

% the outputs in the local coordinate frame are initialized in [0 0 0],
% therefore their first index is not assigned to anything but kept at zero.
Y(2:4) = Y_nominal(2:4) + x(1:3);
X(2:4) = X_nominal(2:4);
theta(2:4) = atan(tan(theta_nominal(2:4)));

end

== matlab function HLB_trp/TrajectoryPlanner/TrajectoryPlanner1/TrajectoryPlanner/MATLAB Function ==
  data: corridor_X input; corridor_Y input; trajectory_segments input; trajectoryPlannerFrame output
function trajectoryPlannerFrame = trajectoryRearrange(corridor_X, corridor_Y, trajectory_segments)

trajectoryPlannerFrame = zeros(3001,2);

n_1 = trajectory_segments(1001);
n_2 = trajectory_segments(2002);
n_3 = trajectory_segments(3003);

trajectoryPlannerFrame(1:n_1,1) = trajectory_segments(1:n_1,1);
trajectoryPlannerFrame(1:n_1,2) = trajectory_segments(1:n_1,2);
trajectoryPlannerFrame(n_1+1:n_1+n_2,1) = trajectory_segments(1002:1001+n_2,1);
trajectoryPlannerFrame(n_1+1:n_1+n_2,2) = trajectory_segments(1002:1001+n_2,2);
trajectoryPlannerFrame(n_1+n_2+1:n_1+n_2+n_3,1) = trajectory_segments(2003:2002+n_3,1);
trajectoryPlannerFrame(n_1+n_2+1:n_1+n_2+n_3,2) = trajectory_segments(2003:2002+n_3,2);


trajectoryPlannerFrame(3001) = n_1 + n_2 + n_3;

if (any(abs(trajectoryPlannerFrame(1:n_1 + n_2 + n_3,2)-corridor_Y(1:n_1 + n_2 + n_3,1)) > 0.1))
    n_1;
end
end

== matlab function HLB_trp/TrajectoryPlanner/TrajectoryPlanner1/TransformationPlannerFrame/corridor_preprocess ==
  data: corridorGlobalFrame input; corridorPlannerFrame output; plannerFrame input
function corridorPlannerFrame  = corridor_preproc(corridorGlobalFrame, plannerFrame)

% function claculates the corridor coordinates in the current planner coordinate system
% outputs:
%   corridorPlannerFrame
%       corridorPlannerFrameX
%       corridorPlannerFrameY
%       corridorPlannerFrameOrientation
%       corridorPlannerFrameCurvature
% inputs:
%   subsegment - subsegment data (500m segment from the current ego position)
%   deltaPos - X, Y, Theta difference between planner frame and nearest ego
%   point
%
% @copyright (C) 2022 Robert Bosch GmbH.
% The reproduction, distribution and utilization of this file as
% well as the communication of its contents to others without express
% authorization is prohibited. Offenders will be held liable for the
% payment of damages. All rights reserved in the event of the grant
% of a patent, utility model or design.
% @version 0.1
% @date 2022-04-20
corridor = corridorGlobalFrame(:,1:2);
corridorPlannerFrame = zeros(301,4);
n = corridorGlobalFrame(301,1);
corridorPlannerFrame(301,1) = n;

T = [cos(plannerFrame(3)) -sin(plannerFrame(3)); sin(plannerFrame(3)) cos(plannerFrame(3))];
corridorPlannerFrame(1:n,1:2) = ([corridor(1:n,1)-plannerFrame(1) corridor(1:n,2) - plannerFrame(2)])*T;
corridorPlannerFrame(1:n,3) = corridorGlobalFrame(1:n,3) - plannerFrame(3);
corridorPlannerFrame(1:n,4) = corridorGlobalFrame(1:n,4);

end

== matlab function HLB_trp/TrajectoryPlanner/TrajectoryPlanner1/TransformationPlannerFrame/MATLAB Function ==
  data: initialized input; retrigger input; egoPoseGlobalFrame input; segmentsParam input; PlannerFrame output; previousPlannerFrame input; trajectoryPreviousPlannerFrame input; anchorPoints input; anchorIndeces input
function PlannerFrame  = get_planner_frame(initialized, retrigger, egoPoseGlobalFrame, segmentsParam, previousPlannerFrame, trajectoryPreviousPlannerFrame, anchorPoints, anchorIndeces)
% Exceptions: no available points behind the vehicle (at least 2 needed)
% points behind us are way too far from the vehicle
% if delta_x is not monotonously increasing then orientation calc failes
% if delta_x is smaller than 10e-8 consider pi/2 or -pi/2 in case of
% delta_y value


if initialized == 0
    PlannerFrame = egoPoseGlobalFrame;
elseif ~retrigger
    PlannerFrame = previousPlannerFrame;
else
    PlannerFrame = zeros(3,1);
    nbAnchorPoints = floor(size(anchorPoints,1)/3);
    n = trajectoryPreviousPlannerFrame(end,1);
    % finding closest point and getting replanCycle (which point is the new
    % planner frame)
    % transforming trajectory from planner frame to global frame
    T = [cos(previousPlannerFrame(3)) -sin(previousPlannerFrame(3)); sin(previousPlannerFrame(3)) cos(previousPlannerFrame(3))];
    
    trajectoryPreviousGlobalFrame = trajectoryPreviousPlannerFrame(1:end-1,:)*T';
    trajectoryPreviousGlobalFrame(:,1) = trajectoryPreviousGlobalFrame(:,1) + previousPlannerFrame(1);
    trajectoryPreviousGlobalFrame(:,2) = trajectoryPreviousGlobalFrame(:,2) + previousPlannerFrame(2);
    distances = ((trajectoryPreviousGlobalFrame(1:n,1)-egoPoseGlobalFrame(1)).^2 + ...
        (trajectoryPreviousGlobalFrame(1:n,2)-egoPoseGlobalFrame(2)).^2).^0.5;
    replanCycle = find(distances == min(distances),1);
    plannerFrameXInPreviousPlannerFrame = trajectoryPreviousPlannerFrame(replanCycle(1,1), 1);
    plannerFrameYInPreviousPlannerFrame = trajectoryPreviousPlannerFrame(replanCycle(1,1), 2);

    % find the relevant segment
    segment_id = find( anchorPoints > PlannerFrame(1), 1 ) - 1;
    if ((segment_id(1,1)==0) ||(segment_id(1,1) > nbAnchorPoints))
        segment_id = nbAnchorPoints-1;
    end

    % get the parameters of selected segments
    c0_selected = segmentsParam(segment_id(1,1), 4);
    c1_selected = segmentsParam(segment_id(1,1), 5);
    theta_0_selected = anchorPoints(2*nbAnchorPoints + segment_id(1,1));

    % calculate arc length for Theta value of planner point
    s_planner = arc_length(trajectoryPreviousPlannerFrame, anchorIndeces(segment_id(1,1)), replanCycle(1,1));

    % Theta calcuation for planner point
    plannerFrameOrientInPreviousPlannerFrame = theta_0_selected + (c0_selected * s_planner) + ((c1_selected / 2) * s_planner * s_planner);

    T_inv =  [cos(previousPlannerFrame(3)) -sin(previousPlannerFrame(3)); sin(previousPlannerFrame(3)) cos(previousPlannerFrame(3))];

    PlannerFrame(1:2) = (T_inv*[plannerFrameXInPreviousPlannerFrame; plannerFrameYInPreviousPlannerFrame]) + ...
        [previousPlannerFrame(1); previousPlannerFrame(2)];
    PlannerFrame(3) = plannerFrameOrientInPreviousPlannerFrame + previousPlannerFrame(3);

    end

end

function [s] = arc_length(previousTrajectory, startIndex, replanCycle)

dx = diff(previousTrajectory(startIndex:replanCycle,1));
dy = diff(previousTrajectory(startIndex:replanCycle,2));
ds = sqrt(dx.*dx + dy.*dy);
s = sum(ds)*0.7109;

end

== matlab function HLB_trp/TrajectoryPlanner/MATLAB Function ==
  data: traj input; trajEgo output; ego input; planner input
function trajEgo = fcn(traj, ego, planner)
trajEgo = zeros(3001,2);

% trajPlanner to trajGlobal
n = traj(3001,1);
trajGlobal = zeros(n,2);
T = [cos(planner(3)) -sin(planner(3)); sin(planner(3)) cos(planner(3))];
trajGlobal(:,:) = [traj(1:n,:)*T'] + [ones(n,1)*planner(1) ones(n,1)*planner(2)];

% trajGlobal to trajEgo
T = [cos(ego(3)) sin(ego(3)); -sin(ego(3)) cos(ego(3))];
trajEgo(1:n,:) = (trajGlobal - [ones(n,1)*ego(1) ones(n,1)*ego(2)])*T';
trajEgo(3001,1) = n;

== matlab function HLB_trp/TrajectoryPlanner/Ego2GlobalFrame ==
  data: corridor_X input; corridorGlobal_X output; corridor_Y input; corridor_c1 input; egoPoseGlobalFrame input; corridorGlobal_Y output; corridorGlobal_c1 output
function [corridorGlobal_X, corridorGlobal_Y, corridorGlobal_c1] = fcn(corridor_X, corridor_Y, corridor_c1, egoPoseGlobalFrame)

    n=corridor_X(301,1);
    corridorGlobal_X = zeros(301,1);
    corridorGlobal_Y = zeros(301,1);
    corridorGlobal_c1 = zeros(301,1);
    corridorGlobal = zeros(301,2);

    T = [cos(egoPoseGlobalFrame(3)) -sin(egoPoseGlobalFrame(3)); sin(egoPoseGlobalFrame(3)) cos(egoPoseGlobalFrame(3))];
    corridorGlobal(1:n,:) = [corridor_X(1:n,1) corridor_Y(1:n,1)]*T' + [ones(n,1)*egoPoseGlobalFrame(1) ones(n,1)*egoPoseGlobalFrame(2)];

    corridorGlobal_X(1:n,1) = corridorGlobal(1:n,1);
    corridorGlobal_Y(1:n,1) = corridorGlobal(1:n,2);
    corridorGlobal_c1(1:n,1) = corridor_c1(1:n,1) + egoPoseGlobalFrame(3);
    
    corridorGlobal_X(301,1) = n;
    corridorGlobal_Y(301,1) = n;
    corridorGlobal_c1(301,1) = n;

end

== matlab function HLB_trp/TrajectoryPlanner/ControlLogic/MATLAB Function ==
  data: corridorGlobal_X input; corridorGlobal_Y input; validity output; egoPoseGlobalFrame input; corridorEgo_X input
function validity = corridorValidity(corridorGlobal_X, corridorGlobal_Y, egoPoseGlobalFrame, corridorEgo_X)

n = corridorGlobal_X(301);
distances = ((corridorGlobal_X(1:n) - egoPoseGlobalFrame(1)).^2 + (corridorGlobal_Y(1:n) - egoPoseGlobalFrame(2)).^2).^0.5;
[invalid_idx] = find(abs(diff(distances)) > 6, 1);

distance_first_point = ((corridorGlobal_X(1) - egoPoseGlobalFrame(1))^2 + (corridorGlobal_Y(1) - egoPoseGlobalFrame(2))^2)^0.5;

% checking monotonity, number of corridor points, distance of first point,
% distance between adjacent points
if ~isempty(invalid_idx) ||  distance_first_point > 5 || ~all(diff(corridorEgo_X(1:n))>0) || n < 2
    validity = false;
else
    validity = true;
end

end

== matlab function HLB_trp/TrajectoryPlanner/MATLAB Function1 ==
  data: corridor_X input; corridorGlobal_X output; corridor_Y input; corridor_c1 input; corridor_c2 input; egoPoseGlobalFrame input; corridorGlobal_Y output; corridorGlobal_c1 output; corridorGlobal_c2 output
function [corridorGlobal_X, corridorGlobal_Y, corridorGlobal_c1, corridorGlobal_c2] = fcn(corridor_X, corridor_Y, corridor_c1, corridor_c2, egoPoseGlobalFrame)

n = corridor_X(301);

if (n >= 2)
    distances_vec = ((corridor_X(1:n) - egoPoseGlobalFrame(1)).^2 + (corridor_Y(1:n) - egoPoseGlobalFrame(2)).^2).^0.5;
    [closest_point_index] = find(distances_vec == min(distances_vec),1);
    closest_point_index = closest_point_index(1);

    corridorGlobal_X = corridor_X(closest_point_index);
    corridorGlobal_Y = corridor_Y(closest_point_index);
    corridorGlobal_c1 = corridor_c1(closest_point_index);
    corridorGlobal_c2 = corridor_c2(closest_point_index);
else
    corridorGlobal_X = 0;
    corridorGlobal_Y = 0;
    corridorGlobal_c1 = 0;
    corridorGlobal_c2 = 0;
end

end

== matlab function HLB_trp/TrajectoryPlanner/MATLAB Function2 ==
  data: trajectoryEgoFrame input; trajectoryGlobalFrame output; egoPoseGlobalFrame input
function trajectoryGlobalFrame = fcn(trajectoryEgoFrame, egoPoseGlobalFrame)

n = trajectoryEgoFrame(3001);
trajectoryGlobalFrame = zeros(3001,2);

R = [cos(egoPoseGlobalFrame(3)) sin(egoPoseGlobalFrame(3));
     -sin(egoPoseGlobalFrame(3)) cos(egoPoseGlobalFrame(3))];
 
traj_rotated = (R' * trajectoryEgoFrame(1:n,:)')';
trajectoryGlobalFrame(1:n,1) = traj_rotated(:,1) + egoPoseGlobalFrame(1);
trajectoryGlobalFrame(1:n,2) = traj_rotated(:,2) + egoPoseGlobalFrame(2);
trajectoryGlobalFrame(3001) = n;
%{
[only_zeros] = find(trajectoryEgoFrame,1);

if ~isempty(only_zeros)

    n = trajectoryEgoFrame(3001);
    trajectoryGlobalFrame = zeros(1,2);
    transformed_traj = zeros(n,2);

    R = [cos(egoPoseGlobalFrame(3)) sin(egoPoseGlobalFrame(3));
        -sin(egoPoseGlobalFrame(3)) cos(egoPoseGlobalFrame(3))];

    traj_rotated = (R' * trajectoryEgoFrame(1:n,:)')';
    transformed_traj(:,1) = traj_rotated(:,1) + egoPoseGlobalFrame(1);
    transformed_traj(:,2) = traj_rotated(:,2) + egoPoseGlobalFrame(2);

    distances_vec = ((transformed_traj(:,1) - egoPoseGlobalFrame(1)).^2 + (transformed_traj(:,2) - egoPoseGlobalFrame(2)).^2).^0.5;
    [closest_point_index] = find(distances_vec == min(distances_vec),1);
    closest_point_index = closest_point_index(1);

    trajectoryGlobalFrame(:,1) = transformed_traj(closest_point_index,1);
    trajectoryGlobalFrame(:,2) = transformed_traj(closest_point_index,2);
else
    trajectoryGlobalFrame = zeros(1,2);
end
%}

end
